simulink model "feng_rx_test"  (R2012b)
settings: Solver=FixedStepDiscrete  SolverMode=SingleTasking  StartTime=0.0  StopTime=10000  RelTol=1e-3
undefined symbols (not defined in the file or in its folder): Down, Up
libraries: xbsIndex_r4 x5664, casper_library_misc x10, casper_library_communications x8, xps_library x3, casper_library_delays x2, simulink x1
(part 9 of 47)

== system feng_rx_test/sync_gen ==
  note: check that 0 timestamps
      | are the correct number of data
      | samples apart
  note: generate sync
      | on last sample of
      | data block
  note: generate single sync pulse
      | on first block edge after
      | a reset or an error
  rst : Inport
  din : Inport  Port=2
  en : Inport  Port=3
  time_in : Inport  Port=4
  Gateway Out{1..10} (10 alike) : xbsIndex_r4/Gateway Out  inherit_from_input=off  hdl_port=on  timing_constraint=None  locs_specified=off  LOCs={}  UseAsDAC=off  DACChannel='1'  block_type=gatewayout
  Logical1 : xbsIndex_r4/Logical  logical_function=XOR  inputs=2  en=off  latency=0  precision=Full  arith_type=Unsigned  n_bits=16  bin_pt=0  align_bp=on  dbl_ovrd=off  block_type=logical
  Logical2 : xbsIndex_r4/Logical  logical_function=OR  inputs=2  en=off  latency=0  precision=Full  arith_type=Unsigned  n_bits=16  bin_pt=0  align_bp=on  dbl_ovrd=off  block_type=logical
  Logical{3..6} (4 alike) : xbsIndex_r4/Logical  logical_function=AND  inputs=2  en=off  latency=0  precision=Full  arith_type=Unsigned  n_bits=16  bin_pt=0  align_bp=on  dbl_ovrd=off  block_type=logical
  Relational : xbsIndex_r4/Relational  mode=a=b  en=off  latency=1  dbl_ovrd=off  block_type=relational
  Relational1 : xbsIndex_r4/Relational  mode=a=b  en=off  latency=0  dbl_ovrd=off  block_type=relational
  Relational3 : xbsIndex_r4/Relational  mode=a=b  en=off  latency=0  dbl_ovrd=off  block_type=relational
  Scope1 : Scope  NumInputPorts=7
      settings: YMin=1.525e+06~-1~-1~-1~1.525e+06~-5~-5  YMax=1.565e+06~1~1~1~1.565e+06~5~5  SaveName=ScopeData3
  Scope2 : Scope  NumInputPorts=3
      settings: YMin=1~0~0  YMax=1~1~1  SaveName=ScopeData4
  constant : xbsIndex_r4/Constant  const=0  gui_display_data_type=Fixed-point  arith_type=Unsigned  n_bits=(n_bits_frequencies - n_bits_streams) + n_bits_packet_size + 1  bin_pt=0  preci_type=Single  exp_width=8  frac_width=24  explicit_period=on  period=1  equ=P=C  opselect=C  inp2=PCIN>>17  opr=+  inp1=P  carry=CIN  dbl_ovrd=off  block_type=constant
  constant1 : xbsIndex_r4/Constant  const=0  gui_display_data_type=Fixed-point  arith_type=Unsigned  n_bits=(n_bits_frequencies - n_bits_streams) + n_bits_packet_size + 1  bin_pt=0  preci_type=Single  exp_width=8  frac_width=24  explicit_period=on  period=1  equ=P=C  opselect=C  inp2=PCIN>>17  opr=+  inp1=P  carry=CIN  dbl_ovrd=off  block_type=constant
  counter : xbsIndex_r4/Counter  cnt_type=Count Limited  cnt_to=2^((n_bits_frequencies - n_bits_streams) + n_bits_packet_size + 1 + n_bits_count) * (reorder_order*unscrambler_order) - 2^n_bits_count  operation=Up  start_count=0  cnt_by_val=2^n_bits_count  arith_type=Unsigned  n_bits=(n_bits_frequencies - n_bits_streams) + n_bits_packet_size + 1 + ceil(log2(reorder_order*unscrambler_order)) + n_bits_count  bin_pt=0  load_pin=off  rst=on  en=on  explicit_period=on  period=1  dbl_ovrd=off  use_behavioral_HDL=off  implementation=Fabric  block_type=counter
  ddin{0..2,4} (4 alike) : xbsIndex_r4/Delay  rst=off  infoeditControl=Selection of Reset will increase slice count due to use of real FFs and instead of SRLs  en=off  latency=1  dbl_ovrd=off  reg_retiming=on  block_type=delay
  ddin3 : xbsIndex_r4/Delay  rst=off  infoeditControl=Selection of Reset will increase slice count due to use of real FFs and instead of SRLs  en=on  latency=2  dbl_ovrd=off  reg_retiming=on  block_type=delay
  dedge0 : xbsIndex_r4/Delay  rst=off  infoeditControl=Selection of Reset will increase slice count due to use of real FFs and instead of SRLs  en=off  latency=1  dbl_ovrd=off  reg_retiming=on  block_type=delay
  dedge1 : xbsIndex_r4/Delay  rst=off  infoeditControl=Selection of Reset will increase slice count due to use of real FFs and instead of SRLs  en=off  latency=1  dbl_ovrd=off  reg_retiming=on  block_type=delay
  dedge2 : xbsIndex_r4/Delay  rst=on  infoeditControl=Selection of Reset will increase slice count due to use of real FFs and instead of SRLs  en=on  latency=1  dbl_ovrd=off  reg_retiming=off  block_type=delay
  den{0..4} (5 alike) : xbsIndex_r4/Delay  rst=off  infoeditControl=Selection of Reset will increase slice count due to use of real FFs and instead of SRLs  en=off  latency=1  dbl_ovrd=off  reg_retiming=on  block_type=delay
  derr : xbsIndex_r4/Delay  rst=off  infoeditControl=Selection of Reset will increase slice count due to use of real FFs and instead of SRLs  en=off  latency=1  dbl_ovrd=off  reg_retiming=on  block_type=delay
  dsync : xbsIndex_r4/Delay  rst=off  infoeditControl=Selection of Reset will increase slice count due to use of real FFs and instead of SRLs  en=off  latency=1  dbl_ovrd=off  reg_retiming=on  block_type=delay
  dtime{0..2,4} (4 alike) : xbsIndex_r4/Delay  rst=off  infoeditControl=Selection of Reset will increase slice count due to use of real FFs and instead of SRLs  en=off  latency=1  dbl_ovrd=off  reg_retiming=on  block_type=delay
  dtime3 : xbsIndex_r4/Delay  rst=off  infoeditControl=Selection of Reset will increase slice count due to use of real FFs and instead of SRLs  en=on  latency=2  dbl_ovrd=off  reg_retiming=on  block_type=delay
  edge_detect : Subsystem  AncestorBlock=casper_library_misc/edge_detect  mask(edge_detect){edge=Rising, polarity=Active High, x_in=[0 0.08 0.08 0.16 0.16 0.24 0.24 0.32 0.32 0.4], y_in=[-1 -1  1  1  1  1  1  1  1  1], x_out=[0.6 0.68 0.68 0.76 0.76 0.84 0.84 0.92 0.92 1], y_out=[-1 -1  1  1 -1 -1 -1 -1 -1 -1]}
      mask prompts: edge "Edge Type"; polarity "Output Polarity"; x_in "Input X Positions"; y_in "Input Y Positions"; x_out "Output X Positions"; y_out "Output Y Positions"
      mask help: Output is active for one-cycle after each edge of the specified type (i.e. rising, falling or both).
      mask init: same as feng_rx_test/edge_detect
      settings: AttributesFormatString=|
      | rising edges
      | active high
      mask Help: Output is active for one-cycle after each edge of the specified type (i.e. rising, falling, or both).  Latency is zero.
      mask TypeOptions edge: Rising | Falling | Both
      mask TypeOptions polarity: Active High | Active Low
      mask Display:
      | plot(x_in_num,0.5+y_in_num*0.2);
      | plot(x_out_num,0.5+y_out_num*0.2);
  edge_detect1 : Subsystem  AncestorBlock=casper_library_misc/edge_detect  mask(edge_detect){edge=Rising, polarity=Active High, x_in=[0 0.08 0.08 0.16 0.16 0.24 0.24 0.32 0.32 0.4], y_in=[-1 -1  1  1  1  1  1  1  1  1], x_out=[0.6 0.68 0.68 0.76 0.76 0.84 0.84 0.92 0.92 1], y_out=[-1 -1  1  1 -1 -1 -1 -1 -1 -1]}
      mask prompts: edge "Edge Type"; polarity "Output Polarity"; x_in "Input X Positions"; y_in "Input Y Positions"; x_out "Output X Positions"; y_out "Output Y Positions"
      mask help: Output is active for one-cycle after each edge of the specified type (i.e. rising, falling or both).
      mask init: same as feng_rx_test/edge_detect
      settings: AttributesFormatString=|
      | rising edges
      | active high
      mask Help: Output is active for one-cycle after each edge of the specified type (i.e. rising, falling, or both).  Latency is zero.
      mask TypeOptions edge: Rising | Falling | Both
      mask TypeOptions polarity: Active High | Active Low
      mask Display:
      | plot(x_in_num,0.5+y_in_num*0.2);
      | plot(x_out_num,0.5+y_out_num*0.2);
  first : xbsIndex_r4/Delay  rst=on  infoeditControl=Selection of Reset will increase slice count due to use of real FFs and instead of SRLs  en=on  latency=1  dbl_ovrd=off  reg_retiming=on  block_type=delay
  locked : xbsIndex_r4/Delay  rst=off  infoeditControl=Selection of Reset will increase slice count due to use of real FFs and instead of SRLs  en=on  latency=1  dbl_ovrd=off  reg_retiming=on  block_type=delay
  lsbs_count : xbsIndex_r4/Slice  nbits=(n_bits_frequencies - n_bits_streams) + n_bits_packet_size + 1  boolean_output=off  mode=Lower Bit Location + Width  bit1=0  base1=MSB of Input  bit0=0  base0=LSB of Input  dbl_ovrd=off  block_type=slice
  lsbs_timestamp : xbsIndex_r4/Slice  nbits=(n_bits_frequencies - n_bits_streams) + n_bits_packet_size + 1  boolean_output=off  mode=Lower Bit Location + Width  bit1=0  base1=MSB of Input  bit0=0  base0=LSB of Input  dbl_ovrd=off  block_type=slice
  sample_count : xbsIndex_r4/Constant  const=0  gui_display_data_type=Fixed-point  arith_type=Unsigned  n_bits=(n_bits_frequencies - n_bits_streams) + n_bits_packet_size + 1 + ceil(log2(reorder_order*unscrambler_order)) + n_bits_count  bin_pt=0  preci_type=Single  exp_width=8  frac_width=24  explicit_period=on  period=1  equ=P=C  opselect=C  inp2=PCIN>>17  opr=+  inp1=P  carry=CIN  dbl_ovrd=off  block_type=constant
  sync : Outport
  dout : Outport  Port=2
  dvalid : Outport  Port=3
  time_out : Outport  Port=4
  error : Outport  Port=5
  wires:
  en/1 -> den0/1, first/1, first/3
  din/1 -> ddin0/1
  constant/1 -> Relational/2
  time_in/1 -> lsbs_timestamp/1, dtime0/1
  locked/1 -> edge_detect/1(in), Logical4/1, Gateway Out8/1
  ddin0/1 -> ddin4/1
  dtime0/1 -> dtime4/1
  first/1 -> locked/1, Gateway Out6/1
  edge_detect/1(out) -> counter/1
  sample_count/1 -> Relational1/2
  counter/1 -> Relational1/1, Gateway Out3/1, lsbs_count/1
  Relational1/1 -> Logical3/1
  dtime3/1 -> time_out/1
  den3/1 -> dvalid/1
  ddin3/1 -> dout/1
  lsbs_count/1 -> Relational3/1
  constant1/1 -> Relational3/2
  Logical1/1 -> derr/1, Gateway Out9/1, Logical2/2
  derr/1 -> error/1
  rst/1 -> Logical2/1
  Gateway Out3/1 -> Scope1/1
  Gateway Out4/1 -> Scope1/2
  Gateway Out5/1 -> Scope1/3
  Gateway Out6/1 -> Scope2/1
  Gateway Out7/1 -> Scope2/2
  Gateway Out8/1 -> Scope2/3
  Logical2/1 -> Logical4/2
  Logical4/1 -> first/2
  Gateway Out9/1 -> Scope1/4
  lsbs_timestamp/1 -> Relational/1
  Relational3/1 -> Logical6/2
  dedge2/1 -> Logical5/1
  Gateway Out1/1 -> Scope1/5
  Logical6/1 -> Logical1/1, Gateway Out4/1
  Logical5/1 -> Logical1/2, Gateway Out5/1, dedge2/2
  Logical3/1 -> dsync/1
  den0/1 -> den4/1
  dtime2/1 -> dtime3/1, Gateway Out1/1
  ddin2/1 -> Gateway Out2/1, ddin3/1
  den2/1 -> Gateway Out10/1, ddin3/2, dtime3/2, den3/1, Logical3/2, Logical6/1, Logical5/2, counter/2
  den1/1 -> den2/1
  ddin1/1 -> ddin2/1
  dtime1/1 -> dtime2/1
  dedge1/1 -> dedge2/1, dedge2/3
  dsync/1 -> sync/1
  ddin4/1 -> ddin1/1
  den4/1 -> den1/1
  dtime4/1 -> dtime1/1
  Relational/1 -> edge_detect1/1(in)
  dedge0/1 -> dedge1/1, locked/2, Gateway Out7/1
  Gateway Out10/1 -> Scope1/6
  Gateway Out2/1 -> Scope1/7
  edge_detect1/1(out) -> dedge0/1

== system feng_rx_test/tx_metadata ==
  sim_1 : Inport
  sim_2 : Inport  Port=2
  convert1_1 : DataTypeConversion  OutDataTypeStr=fixdt('ufix16_En0')  LockScale=on
  convert1_2 : DataTypeConversion  OutDataTypeStr=fixdt('ufix16_En0')  LockScale=on
  convert2_1 : DataTypeConversion  OutDataTypeStr=fixdt('ufix16_En0')  ConvertRealWorld=Stored Integer (SI)  LockScale=on
  convert2_2 : DataTypeConversion  OutDataTypeStr=fixdt('ufix16_En0')  ConvertRealWorld=Stored Integer (SI)  LockScale=on
  feng_rx_test_tx_metadata_user_data_out : xbsIndex_r4/Gateway In  gui_display_data_type=Fixed-point  arith_type=Unsigned  n_bits=32  bin_pt=0  preci_type=Single  exp_width=8  frac_width=24  quantization="Round  (unbiased: +/- Inf)"  overflow=Saturate  period=1  dbl_ovrd=off  timing_constraint=None  locs_specified=off  LOCs={}  UseAsADC=off  ADCChannel='1'  inherit_from_input=off  hdl_port=on  block_type=gatewayin
  gain_1 : Gain  Gain=65536
  gain_2 : Gain
  io_delay : xbsIndex_r4/Delay  rst=off  infoeditControl=Selection of Reset will increase slice count due to use of real FFs and instead of SRLs  en=off  latency=0  dbl_ovrd=off  reg_retiming=on  block_type=delay
  reint1 : xbsIndex_r4/Reinterpret  force_arith_type=on  arith_type=Unsigned  force_bin_pt=on  bin_pt=0  block_type=reinterpret
  reint2 : xbsIndex_r4/Reinterpret  force_arith_type=on  arith_type=Unsigned  force_bin_pt=on  bin_pt=0  block_type=reinterpret
  sim_add : Sum  OutDataTypeStr=uint32
  slice_board_id : xbsIndex_r4/Slice  nbits=16  boolean_output=off  mode=Lower Bit Location + Width  bit1=0  base1=MSB of Input  bit0=0  base0=LSB of Input  dbl_ovrd=off  block_type=slice
  slice_porttx : xbsIndex_r4/Slice  nbits=16  boolean_output=off  mode=Lower Bit Location + Width  bit1=0  base1=MSB of Input  bit0=16  base0=LSB of Input  dbl_ovrd=off  block_type=slice
  in_porttx : Outport
  in_board_id : Outport  Port=2
  wires:
  feng_rx_test_tx_metadata_user_data_out/1 -> io_delay/1
  sim_add/1 -> feng_rx_test_tx_metadata_user_data_out/1
  sim_1/1 -> convert1_1/1
  convert1_1/1 -> convert2_1/1
  convert2_1/1 -> gain_1/1
  gain_1/1 -> sim_add/1
  io_delay/1 -> slice_porttx/1, slice_board_id/1
  slice_porttx/1 -> reint1/1
  reint1/1 -> in_porttx/1
  sim_2/1 -> convert1_2/1
  convert1_2/1 -> convert2_2/1
  convert2_2/1 -> gain_2/1
  gain_2/1 -> sim_add/2
  slice_board_id/1 -> reint2/1
  reint2/1 -> in_board_id/1

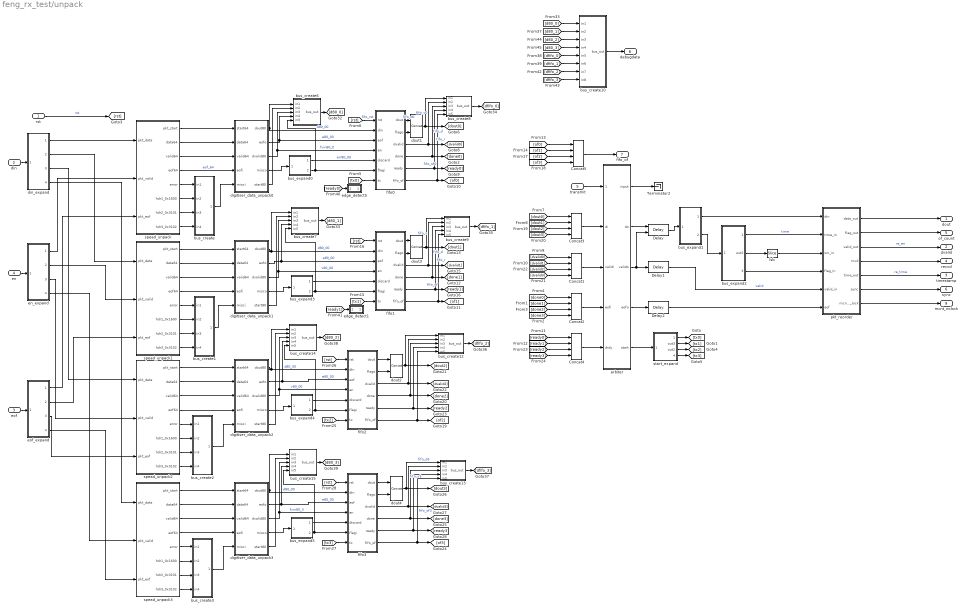
== system feng_rx_test/unpack ==
  rst : Inport
  din : Inport  Port=2
  eof : Inport  Port=3
  en : Inport  Port=4
  transmit : Inport  Port=5
  Concat{1..5} (5 alike) : xbsIndex_r4/Concat  num_inputs=4  dbl_ovrd=off  block_type=concat
  Delay : xbsIndex_r4/Delay  rst=off  infoeditControl=Selection of Reset will increase slice count due to use of real FFs and instead of SRLs  en=on  latency=1  dbl_ovrd=off  reg_retiming=on  block_type=delay
  Delay1 : xbsIndex_r4/Delay  rst=off  infoeditControl=Selection of Reset will increase slice count due to use of real FFs and instead of SRLs  en=off  latency=1  dbl_ovrd=off  reg_retiming=on  block_type=delay
  Delay2 : xbsIndex_r4/Delay  rst=off  infoeditControl=Selection of Reset will increase slice count due to use of real FFs and instead of SRLs  en=off  latency=1  dbl_ovrd=off  reg_retiming=on  block_type=delay
  Terminator2 : Terminator
  arbiter : Subsystem  mask{n_inputs=4, n_bits_input=160 + n_bits_timestamp + n_bits_source + n_bits_of_count, mux_latency=1, preempt=1, n_bits_block_size=n_bits_packet_size-1, n_cycles_preempt=6}
      mask prompts: n_inputs "number of inputs"; n_bits_input "input bit widths"; mux_latency "mux latency"; preempt "preempt start of next block"; n_bits_block_size "data block size (2^?)"; n_cycles_preempt "clock cycles to preempt at"
      mask init:
      | set_param([gcb, '/eofi_mux'], ...
      |     'n_bits', 'ones(1, n_inputs)', ...
      |     'mux_latency', 'mux_latency', ...
      |     'cmplx', 'off', 'misc', 'off');
      | set_param([gcb, '/di_mux'], ...
      |     'n_bits', 'repmat(n_bits_input, 1, n_inputs)', ...
      |     'mux_latency', 'mux_latency', ...
      |     'cmplx', 'off', 'misc', 'off');
      | set_param([gcb, '/validi_mux'], ...
      |     'n_bits', 'ones(1, n_inputs)', ...
      |     'mux_latency', 'mux_latency', ...
      |     'cmplx', 'off', 'misc', 'off');
      | set_param([gcb, '/busy_edge_rep'], ...
      |     'replication', 'n_inputs', ...
      |     'misc', 'off');
  bus_create : Subsystem  AncestorBlock=casper_library_flow_control/bus_create  mask(bus_create){inputNum=4}
      mask prompts: inputNum "Number of inputs:"
      mask init:
      | bus_create_init(gcb,...
      |     'inputNum', inputNum);
  bus_create1 : Subsystem  AncestorBlock=casper_library_flow_control/bus_create  mask(bus_create){inputNum=4}
      mask prompts: inputNum "Number of inputs:"
      mask init:
      | bus_create_init(gcb,...
      |     'inputNum', inputNum);
  bus_create10 : Subsystem  AncestorBlock=casper_library_flow_control/bus_create  mask(bus_create){inputNum=8}
      mask prompts: inputNum "Number of inputs:"
      mask init:
      | bus_create_init(gcb,...
      |     'inputNum', inputNum);
  bus_create12 : Subsystem  AncestorBlock=casper_library_flow_control/bus_create  mask(bus_create){inputNum=5}
      mask prompts: inputNum "Number of inputs:"
      mask init:
      | bus_create_init(gcb,...
      |     'inputNum', inputNum);
  bus_create13 : Subsystem  AncestorBlock=casper_library_flow_control/bus_create  mask(bus_create){inputNum=5}
      mask prompts: inputNum "Number of inputs:"
      mask init:
      | bus_create_init(gcb,...
      |     'inputNum', inputNum);
  bus_create14 : Subsystem  AncestorBlock=casper_library_flow_control/bus_create  mask(bus_create){inputNum=5}
      mask prompts: inputNum "Number of inputs:"
      mask init:
      | bus_create_init(gcb,...
      |     'inputNum', inputNum);
  bus_create15 : Subsystem  AncestorBlock=casper_library_flow_control/bus_create  mask(bus_create){inputNum=5}
      mask prompts: inputNum "Number of inputs:"
      mask init:
      | bus_create_init(gcb,...
      |     'inputNum', inputNum);
  bus_create2 : Subsystem  AncestorBlock=casper_library_flow_control/bus_create  mask(bus_create){inputNum=4}
      mask prompts: inputNum "Number of inputs:"
      mask init:
      | bus_create_init(gcb,...
      |     'inputNum', inputNum);
  bus_create3 : Subsystem  AncestorBlock=casper_library_flow_control/bus_create  mask(bus_create){inputNum=4}
      mask prompts: inputNum "Number of inputs:"
      mask init:
      | bus_create_init(gcb,...
      |     'inputNum', inputNum);
  bus_create6 : Subsystem  AncestorBlock=casper_library_flow_control/bus_create  mask(bus_create){inputNum=5}
      mask prompts: inputNum "Number of inputs:"
      mask init:
      | bus_create_init(gcb,...
      |     'inputNum', inputNum);
  bus_create7 : Subsystem  AncestorBlock=casper_library_flow_control/bus_create  mask(bus_create){inputNum=5}
      mask prompts: inputNum "Number of inputs:"
      mask init:
      | bus_create_init(gcb,...
      |     'inputNum', inputNum);
  bus_create8 : Subsystem  AncestorBlock=casper_library_flow_control/bus_create  mask(bus_create){inputNum=5}
      mask prompts: inputNum "Number of inputs:"
      mask init:
      | bus_create_init(gcb,...
      |     'inputNum', inputNum);
  bus_create9 : Subsystem  AncestorBlock=casper_library_flow_control/bus_create  mask(bus_create){inputNum=5}
      mask prompts: inputNum "Number of inputs:"
      mask init:
      | bus_create_init(gcb,...
      |     'inputNum', inputNum);
  bus_expand0 : Subsystem  AncestorBlock=casper_library_flow_control/bus_expand  mask(bus_expand){mode=divisions of arbitrary size, outputNum=1, outputWidth=[1, sum([n_bits_timestamp, n_bits_source, n_bits_of_count])], outputBinaryPt=[0 0], outputArithmeticType=[2 0], show_format=on, outputToWorkspace=off, variablePrefix=out, outputToModelAsWell=on}
      mask prompts: outputNum "Number of outputs:"; outputWidth "Output width [msb ... lsb]:"; outputBinaryPt "Output binary point position [msb ... lsb]:"; outputArithmeticType "Output arithmetic type (ufix=0, fix=1, bool=2) [msb ... lsb]:"; show_format "Print format string?"; outputToWorkspace "Output to workspace?"; variablePrefix "Variable name prefix:"; outputToModelAsWell "Output to model as well?"
      mask help:
      | Expands a 'bus' made using a bus_create or Xilinx
      | concat block.
      | The input will be divided into the specified number
      | of outputs with the specified arithmetic types.
      | Divisions are made from most significant bit.
      mask init: same as feng_rx_test/bus_expand11
      settings: AttributesFormatString=2 outputs: b,uf144.0,
      mask TypeOptions mode: divisions of equal size | divisions of arbitrary size
      mask Callback mode: bus_expand_callback();
      mask Callback outputWidth: bus_expand_callback();
      mask Callback outputToWorkspace: bus_expand_callback();
  bus_expand1 : Subsystem  AncestorBlock=casper_library_flow_control/bus_expand  mask(bus_expand){mode=divisions of arbitrary size, outputNum=1, outputWidth=[160, sum([n_bits_timestamp, n_bits_source, n_bits_of_count])], outputBinaryPt=[0 0], outputArithmeticType=[0 0], show_format=off, outputToWorkspace=off, variablePrefix=out, outputToModelAsWell=on}
      mask prompts: outputNum "Number of outputs:"; outputWidth "Output width [msb ... lsb]:"; outputBinaryPt "Output binary point position [msb ... lsb]:"; outputArithmeticType "Output arithmetic type (ufix=0, fix=1, bool=2) [msb ... lsb]:"; show_format "Print format string?"; outputToWorkspace "Output to workspace?"; variablePrefix "Variable name prefix:"; outputToModelAsWell "Output to model as well?"
      mask help:
      | Expands a 'bus' made using a bus_create or Xilinx
      | concat block.
      | The input will be divided into the specified number
      | of outputs with the specified arithmetic types.
      | Divisions are made from most significant bit.
      mask init: same as feng_rx_test/bus_expand11
      settings: AttributesFormatString=2 outputs
      mask TypeOptions mode: divisions of equal size | divisions of arbitrary size
      mask Callback mode: bus_expand_callback();
      mask Callback outputWidth: bus_expand_callback();
      mask Callback outputToWorkspace: bus_expand_callback();
  bus_expand2 : Subsystem  AncestorBlock=casper_library_flow_control/bus_expand  mask(bus_expand){mode=divisions of arbitrary size, outputNum=1, outputWidth=[n_bits_timestamp, n_bits_source, n_bits_of_count], outputBinaryPt=[0 0 0], outputArithmeticType=[0 0 0], show_format=off, outputToWorkspace=off, variablePrefix=out, outputToModelAsWell=on}
      mask prompts: outputNum "Number of outputs:"; outputWidth "Output width [msb ... lsb]:"; outputBinaryPt "Output binary point position [msb ... lsb]:"; outputArithmeticType "Output arithmetic type (ufix=0, fix=1, bool=2) [msb ... lsb]:"; show_format "Print format string?"; outputToWorkspace "Output to workspace?"; variablePrefix "Variable name prefix:"; outputToModelAsWell "Output to model as well?"
      mask help:
      | Expands a 'bus' made using a bus_create or Xilinx
      | concat block.
      | The input will be divided into the specified number
      | of outputs with the specified arithmetic types.
      | Divisions are made from most significant bit.
      mask init: same as feng_rx_test/bus_expand11
      settings: AttributesFormatString=3 outputs
      mask TypeOptions mode: divisions of equal size | divisions of arbitrary size
      mask Callback mode: bus_expand_callback();
      mask Callback outputWidth: bus_expand_callback();
      mask Callback outputToWorkspace: bus_expand_callback();
  bus_expand3 : Subsystem  AncestorBlock=casper_library_flow_control/bus_expand  mask(bus_expand){mode=divisions of arbitrary size, outputNum=1, outputWidth=[1, sum([n_bits_timestamp, n_bits_source, n_bits_of_count])], outputBinaryPt=[0 0], outputArithmeticType=[2 0], show_format=off, outputToWorkspace=off, variablePrefix=out, outputToModelAsWell=on}
      mask prompts: outputNum "Number of outputs:"; outputWidth "Output width [msb ... lsb]:"; outputBinaryPt "Output binary point position [msb ... lsb]:"; outputArithmeticType "Output arithmetic type (ufix=0, fix=1, bool=2) [msb ... lsb]:"; show_format "Print format string?"; outputToWorkspace "Output to workspace?"; variablePrefix "Variable name prefix:"; outputToModelAsWell "Output to model as well?"
      mask help:
      | Expands a 'bus' made using a bus_create or Xilinx
      | concat block.
      | The input will be divided into the specified number
      | of outputs with the specified arithmetic types.
      | Divisions are made from most significant bit.
      mask init: same as feng_rx_test/bus_expand11
      settings: AttributesFormatString=2 outputs
      mask TypeOptions mode: divisions of equal size | divisions of arbitrary size
      mask Callback mode: bus_expand_callback();
      mask Callback outputWidth: bus_expand_callback();
      mask Callback outputToWorkspace: bus_expand_callback();
  bus_expand4 : Subsystem  AncestorBlock=casper_library_flow_control/bus_expand  mask(bus_expand){mode=divisions of arbitrary size, outputNum=1, outputWidth=[1, sum([n_bits_timestamp, n_bits_source, n_bits_of_count])], outputBinaryPt=[0 0], outputArithmeticType=[2 0], show_format=off, outputToWorkspace=off, variablePrefix=out, outputToModelAsWell=on}
      mask prompts: outputNum "Number of outputs:"; outputWidth "Output width [msb ... lsb]:"; outputBinaryPt "Output binary point position [msb ... lsb]:"; outputArithmeticType "Output arithmetic type (ufix=0, fix=1, bool=2) [msb ... lsb]:"; show_format "Print format string?"; outputToWorkspace "Output to workspace?"; variablePrefix "Variable name prefix:"; outputToModelAsWell "Output to model as well?"
      mask help:
      | Expands a 'bus' made using a bus_create or Xilinx
      | concat block.
      | The input will be divided into the specified number
      | of outputs with the specified arithmetic types.
      | Divisions are made from most significant bit.
      mask init: same as feng_rx_test/bus_expand11
      settings: AttributesFormatString=2 outputs
      mask TypeOptions mode: divisions of equal size | divisions of arbitrary size
      mask Callback mode: bus_expand_callback();
      mask Callback outputWidth: bus_expand_callback();
      mask Callback outputToWorkspace: bus_expand_callback();
  bus_expand5 : Subsystem  AncestorBlock=casper_library_flow_control/bus_expand  mask(bus_expand){mode=divisions of arbitrary size, outputNum=1, outputWidth=[1, sum([n_bits_timestamp, n_bits_source, n_bits_of_count])], outputBinaryPt=[0 0], outputArithmeticType=[2 0], show_format=off, outputToWorkspace=off, variablePrefix=out, outputToModelAsWell=on}
      mask prompts: outputNum "Number of outputs:"; outputWidth "Output width [msb ... lsb]:"; outputBinaryPt "Output binary point position [msb ... lsb]:"; outputArithmeticType "Output arithmetic type (ufix=0, fix=1, bool=2) [msb ... lsb]:"; show_format "Print format string?"; outputToWorkspace "Output to workspace?"; variablePrefix "Variable name prefix:"; outputToModelAsWell "Output to model as well?"
      mask help:
      | Expands a 'bus' made using a bus_create or Xilinx
      | concat block.
      | The input will be divided into the specified number
      | of outputs with the specified arithmetic types.
      | Divisions are made from most significant bit.
      mask init: same as feng_rx_test/bus_expand11
      settings: AttributesFormatString=2 outputs
      mask TypeOptions mode: divisions of equal size | divisions of arbitrary size
      mask Callback mode: bus_expand_callback();
      mask Callback outputWidth: bus_expand_callback();
      mask Callback outputToWorkspace: bus_expand_callback();
  digitiser_data_unpack0 : Subsystem
  digitiser_data_unpack1 : Subsystem
  digitiser_data_unpack2 : Subsystem
  digitiser_data_unpack3 : Subsystem
  din_expand : Subsystem  AncestorBlock=casper_library_flow_control/bus_expand  mask(bus_expand){mode=divisions of equal size, outputNum=4, outputWidth=64, outputBinaryPt=0, outputArithmeticType=0, show_format=off, outputToWorkspace=off, variablePrefix=out, outputToModelAsWell=on}
      mask prompts: outputNum "Number of outputs:"; outputWidth "Output width:"; outputBinaryPt "Output binary point position:"; outputArithmeticType "Output arithmetic type (ufix=0, fix=1, bool=2):"; show_format "Print format string?"; outputToWorkspace "Output to workspace?"; variablePrefix "Variable name prefix:"; outputToModelAsWell "Output to model as well?"
      mask help:
      | Expands a 'bus' made using a bus_create or Xilinx
      | concat block.
      | The input will be divided into the specified number
      | of outputs with the specified arithmetic types.
      | Divisions are made from most significant bit.
      mask init: same as feng_rx_test/bus_expand11
      settings: AttributesFormatString=4 outputs
      mask TypeOptions mode: divisions of equal size | divisions of arbitrary size
      mask Callback mode: bus_expand_callback();
      mask Callback outputWidth: bus_expand_callback();
      mask Callback outputToWorkspace: bus_expand_callback();
  dout{1..4} (4 alike) : xbsIndex_r4/Concat  num_inputs=2  dbl_ovrd=off  block_type=concat
  edge_detect1 : Subsystem  AncestorBlock=casper_library_misc/edge_detect  mask(edge_detect){edge=Rising, polarity=Active High, x_in=[0 0.08 0.08 0.16 0.16 0.24 0.24 0.32 0.32 0.4], y_in=[-1 -1  1  1  1  1  1  1  1  1], x_out=[0.6 0.68 0.68 0.76 0.76 0.84 0.84 0.92 0.92 1], y_out=[-1 -1  1  1 -1 -1 -1 -1 -1 -1]}
      mask prompts: edge "Edge Type"; polarity "Output Polarity"; x_in "Input X Positions"; y_in "Input Y Positions"; x_out "Output X Positions"; y_out "Output Y Positions"
      mask help: Output is active for one-cycle after each edge of the specified type (i.e. rising, falling or both).
      mask init: same as feng_rx_test/edge_detect
      settings: AttributesFormatString=|
      | rising edges
      | active high
      mask Help: Output is active for one-cycle after each edge of the specified type (i.e. rising, falling, or both).  Latency is zero.
      mask TypeOptions edge: Rising | Falling | Both
      mask TypeOptions polarity: Active High | Active Low
      mask Display:
      | plot(x_in_num,0.5+y_in_num*0.2);
      | plot(x_out_num,0.5+y_out_num*0.2);
  edge_detect5 : Subsystem  AncestorBlock=casper_library_misc/edge_detect  mask(edge_detect){edge=Rising, polarity=Active High, x_in=[0 0.08 0.08 0.16 0.16 0.24 0.24 0.32 0.32 0.4], y_in=[-1 -1  1  1  1  1  1  1  1  1], x_out=[0.6 0.68 0.68 0.76 0.76 0.84 0.84 0.92 0.92 1], y_out=[-1 -1  1  1 -1 -1 -1 -1 -1 -1]}
      mask prompts: edge "Edge Type"; polarity "Output Polarity"; x_in "Input X Positions"; y_in "Input Y Positions"; x_out "Output X Positions"; y_out "Output Y Positions"
      mask help: Output is active for one-cycle after each edge of the specified type (i.e. rising, falling or both).
      mask init: same as feng_rx_test/edge_detect
      settings: AttributesFormatString=|
      | rising edges
      | active high
      mask Help: Output is active for one-cycle after each edge of the specified type (i.e. rising, falling, or both).  Latency is zero.
      mask TypeOptions edge: Rising | Falling | Both
      mask TypeOptions polarity: Active High | Active Low
      mask Display:
      | plot(x_in_num,0.5+y_in_num*0.2);
      | plot(x_out_num,0.5+y_out_num*0.2);
  en_expand : Subsystem  AncestorBlock=casper_library_flow_control/bus_expand  mask(bus_expand){mode=divisions of equal size, outputNum=4, outputWidth=1, outputBinaryPt=0, outputArithmeticType=2, show_format=off, outputToWorkspace=off, variablePrefix=out, outputToModelAsWell=on}
      mask prompts: outputNum "Number of outputs:"; outputWidth "Output width:"; outputBinaryPt "Output binary point position:"; outputArithmeticType "Output arithmetic type (ufix=0, fix=1, bool=2):"; show_format "Print format string?"; outputToWorkspace "Output to workspace?"; variablePrefix "Variable name prefix:"; outputToModelAsWell "Output to model as well?"
      mask help:
      | Expands a 'bus' made using a bus_create or Xilinx
      | concat block.
      | The input will be divided into the specified number
      | of outputs with the specified arithmetic types.
      | Divisions are made from most significant bit.
      mask init: same as feng_rx_test/bus_expand11
      settings: AttributesFormatString=4 outputs
      mask TypeOptions mode: divisions of equal size | divisions of arbitrary size
      mask Callback mode: bus_expand_callback();
      mask Callback outputWidth: bus_expand_callback();
      mask Callback outputToWorkspace: bus_expand_callback();
  eof_expand : Subsystem  AncestorBlock=casper_library_flow_control/bus_expand  mask(bus_expand){mode=divisions of equal size, outputNum=4, outputWidth=1, outputBinaryPt=0, outputArithmeticType=2, show_format=off, outputToWorkspace=off, variablePrefix=out, outputToModelAsWell=on}
      mask prompts: outputNum "Number of outputs:"; outputWidth "Output width:"; outputBinaryPt "Output binary point position:"; outputArithmeticType "Output arithmetic type (ufix=0, fix=1, bool=2):"; show_format "Print format string?"; outputToWorkspace "Output to workspace?"; variablePrefix "Variable name prefix:"; outputToModelAsWell "Output to model as well?"
      mask help:
      | Expands a 'bus' made using a bus_create or Xilinx
      | concat block.
      | The input will be divided into the specified number
      | of outputs with the specified arithmetic types.
      | Divisions are made from most significant bit.
      mask init: same as feng_rx_test/bus_expand11
      settings: AttributesFormatString=4 outputs
      mask TypeOptions mode: divisions of equal size | divisions of arbitrary size
      mask Callback mode: bus_expand_callback();
      mask Callback outputWidth: bus_expand_callback();
      mask Callback outputToWorkspace: bus_expand_callback();
  fifo0 : Subsystem  mask{n_bits_din=80, n_bits_flag=sum([n_bits_timestamp, n_bits_source, n_bits_of_count]), scale_factor_bits=1, input_word_count_bits=n_bits_packet_size, bram_latency=bram_latency}
      mask prompts: n_bits_din "input data bit width"; n_bits_flag "flag bit width"; scale_factor_bits "output width scale factor (2^?)"; input_word_count_bits "max input word count (2^?)"; bram_latency "BRAM latency"
  fifo1 : Subsystem  mask{n_bits_din=80, n_bits_flag=sum([n_bits_timestamp, n_bits_source, n_bits_of_count]), scale_factor_bits=1, input_word_count_bits=n_bits_packet_size, bram_latency=bram_latency}
      mask prompts: n_bits_din "input data bit width"; n_bits_flag "flag bit width"; scale_factor_bits "output width scale factor (2^?)"; input_word_count_bits "max input word count (2^?)"; bram_latency "BRAM latency"
  fifo2 : Subsystem  mask{n_bits_din=80, n_bits_flag=sum([n_bits_timestamp, n_bits_source, n_bits_of_count]), scale_factor_bits=1, input_word_count_bits=n_bits_packet_size, bram_latency=bram_latency}
      mask prompts: n_bits_din "input data bit width"; n_bits_flag "flag bit width"; scale_factor_bits "output width scale factor (2^?)"; input_word_count_bits "max input word count (2^?)"; bram_latency "BRAM latency"
  fifo3 : Subsystem  mask{n_bits_din=80, n_bits_flag=sum([n_bits_timestamp, n_bits_source, n_bits_of_count]), scale_factor_bits=1, input_word_count_bits=n_bits_packet_size, bram_latency=bram_latency}
      mask prompts: n_bits_din "input data bit width"; n_bits_flag "flag bit width"; scale_factor_bits "output width scale factor (2^?)"; input_word_count_bits "max input word count (2^?)"; bram_latency "BRAM latency"
  lsb : xbsIndex_r4/Slice  nbits=1  boolean_output=off  mode=Lower Bit Location + Width  bit1=0  base1=MSB of Input  bit0=0  base0=LSB of Input  dbl_ovrd=off  block_type=slice
  pkt_reorder : Subsystem  mask{window_bits=n_bits_buffer, window_size_bits=n_bits_packet_size - 1, n_bits_din=80, n_bits_flag=n_bits_of_count, n_bits_timestamp=n_bits_timestamp}
      mask prompts: window_bits "Number of Windows to Buffer (2^?)"; window_size_bits "Window size (2^?)"; n_bits_din "Data bit width in"; n_bits_flag "Flag bit width in"; n_bits_timestamp "Timestamp bit width"
      mask init:
      | fmtstr = sprintf('Buffer space: 2^%i words', window_bits+window_size_bits);
      | set_param(gcb, 'AttributesFormatString', fmtstr);
      settings: AttributesFormatString=Buffer space: 2^11 words
  spead_unpack : Subsystem  Tag=casper:spead_unpack  AncestorBlock=casper_library_communications/spead_unpack  mask(spead_unpack_mask){payload_length=640, header_ids=[5632 12545 12546], spead_msw=64, spead_lsw=48, spead_version=4, combine_errors=on}
      mask prompts: payload_length "Payload length in 64-bit words"; header_ids "SPEAD header IDs (decimal)"; spead_msw "SPEAD Flavour (MSw)"; spead_lsw "SPEAD Flavour (LSw)"; spead_version "SPEAD version"; combine_errors "Combine error flags"
      mask help: This block receives a 64-bit-word stream that contains a SPEAD stream. It checks the SPEAD headers are being correctly received. It presents the user with all headers on the first valid cycle of data along with a flag to indicate a header or packet-length error.
      mask init:
      | spead_unpack_init(gcb)
  spead_unpack1 : Subsystem  Tag=casper:spead_unpack  AncestorBlock=casper_library_communications/spead_unpack  mask(spead_unpack_mask){payload_length=640, header_ids=[5632 12545 12546], spead_msw=64, spead_lsw=48, spead_version=4, combine_errors=on}
      mask prompts: payload_length "Payload length in 64-bit words"; header_ids "SPEAD header IDs (decimal)"; spead_msw "SPEAD Flavour (MSw)"; spead_lsw "SPEAD Flavour (LSw)"; spead_version "SPEAD version"; combine_errors "Combine error flags"
      mask help: This block receives a 64-bit-word stream that contains a SPEAD stream. It checks the SPEAD headers are being correctly received. It presents the user with all headers on the first valid cycle of data along with a flag to indicate a header or packet-length error.
      mask init:
      | spead_unpack_init(gcb)
  spead_unpack2 : Subsystem  Tag=casper:spead_unpack  AncestorBlock=casper_library_communications/spead_unpack  mask(spead_unpack_mask){payload_length=640, header_ids=[5632 12545 12546], spead_msw=64, spead_lsw=48, spead_version=4, combine_errors=on}
      mask prompts: payload_length "Payload length in 64-bit words"; header_ids "SPEAD header IDs (decimal)"; spead_msw "SPEAD Flavour (MSw)"; spead_lsw "SPEAD Flavour (LSw)"; spead_version "SPEAD version"; combine_errors "Combine error flags"
      mask help: This block receives a 64-bit-word stream that contains a SPEAD stream. It checks the SPEAD headers are being correctly received. It presents the user with all headers on the first valid cycle of data along with a flag to indicate a header or packet-length error.
      mask init:
      | spead_unpack_init(gcb)
  spead_unpack3 : Subsystem  Tag=casper:spead_unpack  AncestorBlock=casper_library_communications/spead_unpack  mask(spead_unpack_mask){payload_length=640, header_ids=[5632 12545 12546], spead_msw=64, spead_lsw=48, spead_version=4, combine_errors=on}
      mask prompts: payload_length "Payload length in 64-bit words"; header_ids "SPEAD header IDs (decimal)"; spead_msw "SPEAD Flavour (MSw)"; spead_lsw "SPEAD Flavour (LSw)"; spead_version "SPEAD version"; combine_errors "Combine error flags"
      mask help: This block receives a 64-bit-word stream that contains a SPEAD stream. It checks the SPEAD headers are being correctly received. It presents the user with all headers on the first valid cycle of data along with a flag to indicate a header or packet-length error.
      mask init:
      | spead_unpack_init(gcb)
  start_expand : Subsystem  AncestorBlock=casper_library_flow_control/bus_expand  mask(bus_expand){mode=divisions of equal size, outputNum=4, outputWidth=1, outputBinaryPt=0, outputArithmeticType=2, show_format=off, outputToWorkspace=off, variablePrefix=out, outputToModelAsWell=on}
      mask prompts: outputNum "Number of outputs:"; outputWidth "Output width:"; outputBinaryPt "Output binary point position:"; outputArithmeticType "Output arithmetic type (ufix=0, fix=1, bool=2):"; show_format "Print format string?"; outputToWorkspace "Output to workspace?"; variablePrefix "Variable name prefix:"; outputToModelAsWell "Output to model as well?"
      mask help:
      | Expands a 'bus' made using a bus_create or Xilinx
      | concat block.
      | The input will be divided into the specified number
      | of outputs with the specified arithmetic types.
      | Divisions are made from most significant bit.
      mask init: same as feng_rx_test/bus_expand11
      settings: AttributesFormatString=4 outputs
      mask TypeOptions mode: divisions of equal size | divisions of arbitrary size
      mask Callback mode: bus_expand_callback();
      mask Callback outputWidth: bus_expand_callback();
      mask Callback outputToWorkspace: bus_expand_callback();
  dout : Outport
  dvalid : Outport  Port=2
  timestamp : Outport  Port=3
  recvd : Outport  Port=4
  of_count : Outport  Port=5
  sync : Outport  Port=6
  fifo_of : Outport  Port=7
  debugdata : Outport  Port=8
  mcnt_nolock : Outport  Port=9
  wires:
  [dfifo_0] -> bus_create10/5(in5)
  [dfifo_3] -> bus_create10/8(in8)
  [dfifo_2] -> bus_create10/7(in7)
  [dfifo_1] -> bus_create10/6(in6)
  [d80_3] -> bus_create10/4(in4)
  [d80_2] -> bus_create10/3(in3)
  [d80_1] -> bus_create10/2(in2)
  [d80_0] -> bus_create10/1(in1)
  digitiser_data_unpack3/5(start80) -> bus_create15/2(in2)
  digitiser_data_unpack2/5(start80) -> bus_create14/2(in2)
  bus_create15/1(bus_out) -> [d80_3]
  bus_create14/1(bus_out) -> [d80_2]
  bus_create13/1(bus_out) -> [dfifo_3]
  bus_create12/1(bus_out) -> [dfifo_2]
  [tx1] -> fifo1/7(tx)
  [tx0] -> fifo0/7(tx)
  pkt_reorder/7(mcnt_no_lock) -> mcnt_nolock/1
  pkt_reorder/6(sync) -> sync/1
  pkt_reorder/5(time_out) -> timestamp/1  "re_time"
  pkt_reorder/4(rcvd) -> recvd/1
  pkt_reorder/3(valid_out) -> dvalid/1  "re_en"
  pkt_reorder/2(flag_out) -> of_count/1
  pkt_reorder/1(data_out) -> dout/1
  [ready1] -> edge_detect1/1(in)
  [ready0] -> edge_detect5/1(in)
  digitiser_data_unpack1/5(start80) -> bus_create7/2(in2)
  bus_create7/1(bus_out) -> [d80_1]
  digitiser_data_unpack0/5(start80) -> bus_create6/2(in2)
  spead_unpack/3(valid64) -> digitiser_data_unpack0/3(valid64)
  spead_unpack/6(hdr1_0x1600) -> bus_create/2(in2)
  bus_create10/1(bus_out) -> debugdata/1
  bus_create9/1(bus_out) -> [dfifo_1]
  bus_create8/1(bus_out) -> [dfifo_0]
  bus_create6/1(bus_out) -> [d80_0]
  fifo0/4(done) -> bus_create8/3(in3), [done0]  "fifo_d"
  dout1/1 -> bus_create8/1(in1), [dout0]
  fifo0/3(dvalid) -> bus_create8/2(in2), [dvalid0]  "fifo_v0"
  fifo0/5(ready) -> bus_create8/4(in4), [ready0]  "fifo_r"
  fifo0/6(fifo_of) -> [of0], bus_create8/5(in5)  "fifo_of0"
  arbiter/5(start) -> start_expand/1(bus_in)
  Concat4/1 -> arbiter/5(drdy)
  Concat2/1 -> arbiter/4(eofi)
  Concat3/1 -> arbiter/2(di)
  Concat1/1 -> arbiter/3(validi)
  transmit/1 -> arbiter/1(transmit)
  start_expand/1(msb_out4) -> [tx0]
  start_expand/2(out3) -> [tx1]
  start_expand/3(out2) -> [tx2]
  start_expand/4(lsb_out1) -> [tx3]
  [done0] -> Concat2/1
  [done3] -> Concat2/4
  [done1] -> Concat2/2
  [done2] -> Concat2/3
  [dout0] -> Concat3/1
  [dout1] -> Concat3/2
  [dvalid0] -> Concat1/1
  [dvalid1] -> Concat1/2
  [ready0] -> Concat4/1
  [ready1] -> Concat4/2
  Concat5/1 -> fifo_of/1
  [dout2] -> Concat3/3
  [dout3] -> Concat3/4
  [dvalid2] -> Concat1/3
  [dvalid3] -> Concat1/4
  [ready2] -> Concat4/3
  [ready3] -> Concat4/4
  arbiter/1(input) -> Terminator2/1
  [of0] -> Concat5/1
  [of1] -> Concat5/2
  [of2] -> Concat5/3
  [of3] -> Concat5/4
  rst/1 -> [rst]  "rst"
  [rst] -> fifo0/1(rst)  "fifo_rst"
  din/1 -> din_expand/1(bus_in)
  en/1 -> en_expand/1(bus_in)
  eof/1 -> eof_expand/1(bus_in)
  digitiser_data_unpack0/1(dout80) -> fifo0/2(din), bus_create6/1(in1)  "d80_00"
  digitiser_data_unpack0/4(misco) -> bus_expand0/1(bus_in)
  digitiser_data_unpack0/2(eofo) -> fifo0/3(eof), bus_create6/4(in4)  "e80_00"
  digitiser_data_unpack0/3(dvalid80) -> fifo0/4(en), bus_create6/3(in3)  "fvin80_0"
  bus_expand1/1(msb_out2) -> pkt_reorder/1(din)
  bus_expand1/2(lsb_out1) -> bus_expand2/1(bus_in)
  bus_expand2/1(msb_out3) -> pkt_reorder/2(time_in)  "time"
  bus_expand2/3(lsb_out1) -> pkt_reorder/4(flag_in)
  spead_unpack/1(pkt_start) -> digitiser_data_unpack0/1(start64)
  spead_unpack1/1(pkt_start) -> digitiser_data_unpack1/1(start64)
  spead_unpack2/1(pkt_start) -> digitiser_data_unpack2/1(start64)
  spead_unpack3/1(pkt_start) -> digitiser_data_unpack3/1(start64)
  spead_unpack/2(data64) -> digitiser_data_unpack0/2(data64)
  spead_unpack/4(eof64) -> digitiser_data_unpack0/4(eofi)  "eof_64"
  bus_create/1(bus_out) -> digitiser_data_unpack0/5(misci)
  bus_expand0/1(msb_out2) -> fifo0/5(discard)  "err80_00"
  bus_expand0/2(lsb_out1) -> fifo0/6(flagi), bus_create6/5(in5)
  spead_unpack1/2(data64) -> digitiser_data_unpack1/2(data64)
  spead_unpack1/3(valid64) -> digitiser_data_unpack1/3(valid64)
  spead_unpack1/4(eof64) -> digitiser_data_unpack1/4(eofi)
  spead_unpack1/5(error) -> bus_create1/1(in1)
  spead_unpack1/6(hdr1_0x1600) -> bus_create1/2(in2)
  spead_unpack1/7(hdr2_0x3101) -> bus_create1/3(in3)
  spead_unpack1/8(hdr3_0x3102) -> bus_create1/4(in4)
  bus_create1/1(bus_out) -> digitiser_data_unpack1/5(misci)
  spead_unpack2/2(data64) -> digitiser_data_unpack2/2(data64)
  spead_unpack2/3(valid64) -> digitiser_data_unpack2/3(valid64)
  spead_unpack2/4(eof64) -> digitiser_data_unpack2/4(eofi)
  spead_unpack2/5(error) -> bus_create2/1(in1)
  spead_unpack2/6(hdr1_0x1600) -> bus_create2/2(in2)
  spead_unpack2/7(hdr2_0x3101) -> bus_create2/3(in3)
  spead_unpack2/8(hdr3_0x3102) -> bus_create2/4(in4)
  bus_create2/1(bus_out) -> digitiser_data_unpack2/5(misci)
  spead_unpack3/2(data64) -> digitiser_data_unpack3/2(data64)
  spead_unpack3/3(valid64) -> digitiser_data_unpack3/3(valid64)
  spead_unpack3/4(eof64) -> digitiser_data_unpack3/4(eofi)
  spead_unpack3/5(error) -> bus_create3/1(in1)
  spead_unpack3/6(hdr1_0x1600) -> bus_create3/2(in2)
  spead_unpack3/7(hdr2_0x3101) -> bus_create3/3(in3)
  spead_unpack3/8(hdr3_0x3102) -> bus_create3/4(in4)
  bus_create3/1(bus_out) -> digitiser_data_unpack3/5(misci)
  [rst] -> fifo1/1(rst)
  digitiser_data_unpack1/1(dout80) -> fifo1/2(din), bus_create7/1(in1)  "d80_00"
  digitiser_data_unpack1/4(misco) -> bus_expand3/1(bus_in)
  digitiser_data_unpack1/2(eofo) -> fifo1/3(eof), bus_create7/4(in4)  "e80_00"
  digitiser_data_unpack1/3(dvalid80) -> fifo1/4(en), bus_create7/3(in3)  "v80_00"
  bus_expand3/1(msb_out2) -> fifo1/5(discard)
  bus_expand3/2(lsb_out1) -> fifo1/6(flagi), bus_create7/5(in5)
  fifo1/3(dvalid) -> bus_create9/2(in2), [dvalid1]  "fifo_v"
  fifo1/4(done) -> bus_create9/3(in3), [done1]  "fifo_d"
  fifo1/5(ready) -> bus_create9/4(in4), [ready1]  "fifo_r"
  fifo1/6(fifo_of) -> [of1], bus_create9/5(in5)  "fifo_of"
  [tx2] -> fifo2/7(tx)
  [rst] -> fifo2/1(rst)
  digitiser_data_unpack2/1(dout80) -> fifo2/2(din), bus_create14/1(in1)  "d80_00"
  digitiser_data_unpack2/4(misco) -> bus_expand4/1(bus_in)
  digitiser_data_unpack2/2(eofo) -> fifo2/3(eof), bus_create14/4(in4)  "e80_00"
  digitiser_data_unpack2/3(dvalid80) -> fifo2/4(en), bus_create14/3(in3)  "v80_00"
  bus_expand4/1(msb_out2) -> fifo2/5(discard)
  bus_expand4/2(lsb_out1) -> fifo2/6(flagi), bus_create14/5(in5)
  fifo2/1(dout) -> dout2/1
  fifo2/2(flago) -> dout2/2
  fifo0/1(dout) -> dout1/1  "fifo_d0"
  fifo0/2(flago) -> dout1/2
  fifo1/1(dout) -> dout3/1
  fifo1/2(flago) -> dout3/2
  dout3/1 -> bus_create9/1(in1), [dout1]
  dout2/1 -> [dout2], bus_create12/1(in1)
  fifo2/3(dvalid) -> [dvalid2], bus_create12/2(in2)
  fifo2/4(done) -> [done2], bus_create12/3(in3)
  fifo2/5(ready) -> [ready2], bus_create12/4(in4)
  fifo2/6(fifo_of) -> [of2], bus_create12/5(in5)
  [tx3] -> fifo3/7(tx)
  [rst] -> fifo3/1(rst)
  digitiser_data_unpack3/1(dout80) -> fifo3/2(din), bus_create15/1(in1)  "d80_00"
  digitiser_data_unpack3/4(misco) -> bus_expand5/1(bus_in)
  digitiser_data_unpack3/2(eofo) -> bus_create15/4(in4), fifo3/3(eof)  "e80_00"
  digitiser_data_unpack3/3(dvalid80) -> fifo3/4(en), bus_create15/3(in3)  "fvin80_3"
  bus_expand5/1(msb_out2) -> fifo3/5(discard)
  bus_expand5/2(lsb_out1) -> fifo3/6(flagi), bus_create15/5(in5)
  fifo3/1(dout) -> dout4/1
  fifo3/2(flago) -> dout4/2
  dout4/1 -> [dout3], bus_create13/1(in1)  "fifo_d3"
  fifo3/3(dvalid) -> [dvalid3], bus_create13/2(in2)  "fifo_v3"
  fifo3/4(done) -> [done3], bus_create13/3(in3)
  fifo3/5(ready) -> [ready3], bus_create13/4(in4)
  fifo3/6(fifo_of) -> [of3], bus_create13/5(in5)  "fifo_of3"
  bus_expand2/2(out2) -> lsb/1
  lsb/1 -> pkt_reorder/3(src_in)
  spead_unpack/5(error) -> bus_create/1(in1)
  spead_unpack/7(hdr2_0x3101) -> bus_create/3(in3)
  spead_unpack/8(hdr3_0x3102) -> bus_create/4(in4)
  din_expand/1(msb_out4) -> spead_unpack/1(pkt_data)
  din_expand/2(out3) -> spead_unpack1/1(pkt_data)
  din_expand/3(out2) -> spead_unpack2/1(pkt_data)
  din_expand/4(lsb_out1) -> spead_unpack3/1(pkt_data)
  en_expand/1(msb_out4) -> spead_unpack/2(pkt_valid)
  en_expand/2(out3) -> spead_unpack1/2(pkt_valid)
  en_expand/3(out2) -> spead_unpack2/2(pkt_valid)
  en_expand/4(lsb_out1) -> spead_unpack3/2(pkt_valid)
  eof_expand/1(msb_out4) -> spead_unpack/3(pkt_eof)
  eof_expand/2(out3) -> spead_unpack1/3(pkt_eof)
  eof_expand/3(out2) -> spead_unpack2/3(pkt_eof)
  eof_expand/4(lsb_out1) -> spead_unpack3/3(pkt_eof)
  arbiter/2(do) -> Delay/1
  arbiter/3(valido) -> Delay1/1, Delay/2
  arbiter/4(eofo) -> Delay2/1
  Delay/1 -> bus_expand1/1(bus_in)
  Delay1/1 -> pkt_reorder/5(valid_in)  "valid"
  Delay2/1 -> pkt_reorder/6(eof)

== system feng_rx_test/ct/bus_expand ==
  bus_in : Inport
  reinterpret{1..4} (4 alike) : xbsIndex_r4/Reinterpret  force_arith_type=on  arith_type=Unsigned  force_bin_pt=on  bin_pt=0  block_type=reinterpret
  slice1 : xbsIndex_r4/Slice  nbits=64  boolean_output=off  mode=Upper Bit Location + Width  bit1=-192  base1=MSB of Input  bit0=0  base0=LSB of Input  dbl_ovrd=off  block_type=slice
  slice2 : xbsIndex_r4/Slice  nbits=64  boolean_output=off  mode=Upper Bit Location + Width  bit1=-128  base1=MSB of Input  bit0=0  base0=LSB of Input  dbl_ovrd=off  block_type=slice
  slice3 : xbsIndex_r4/Slice  nbits=64  boolean_output=off  mode=Upper Bit Location + Width  bit1=-64  base1=MSB of Input  bit0=0  base0=LSB of Input  dbl_ovrd=off  block_type=slice
  slice4 : xbsIndex_r4/Slice  nbits=64  boolean_output=off  mode=Upper Bit Location + Width  bit1=0  base1=MSB of Input  bit0=0  base0=LSB of Input  dbl_ovrd=off  block_type=slice
  msb_out4 : Outport
  out3 : Outport  Port=2
  out2 : Outport  Port=3
  lsb_out1 : Outport  Port=4
  wires:
  reinterpret1/1 -> lsb_out1/1
  slice1/1 -> reinterpret1/1
  reinterpret2/1 -> out2/1
  slice2/1 -> reinterpret2/1
  reinterpret3/1 -> out3/1
  slice3/1 -> reinterpret3/1
  reinterpret4/1 -> msb_out4/1
  slice4/1 -> reinterpret4/1
  bus_in/1 -> slice1/1, slice2/1, slice3/1, slice4/1
